simulink model "Redresseur_MLI_3Ph_MLI_antiwindup_sign"  (R2018b)
settings: Solver=ode8  StartTime=0.0  StopTime=Ts  FixedStep=1e-6  RelTol=1e-3
undefined symbols (not defined in the file): C, Im, inverter_matrix, K, L, R, Ta, Td, Ti, V
libraries: simulink x1
settings Model: Creator=driss  LastModifiedBy=driss
settings DataIOCC: ReturnWorkspaceOutputs=on
settings DebuggingCC: UnconnectedInputMsg=none  UnconnectedOutputMsg=none  UnconnectedLineMsg=none
settings ModelReferenceCC: EnableRefExpFcnMdlSchedulingChecks=off
settings RTWCC: Description=Generic Real-Time Target

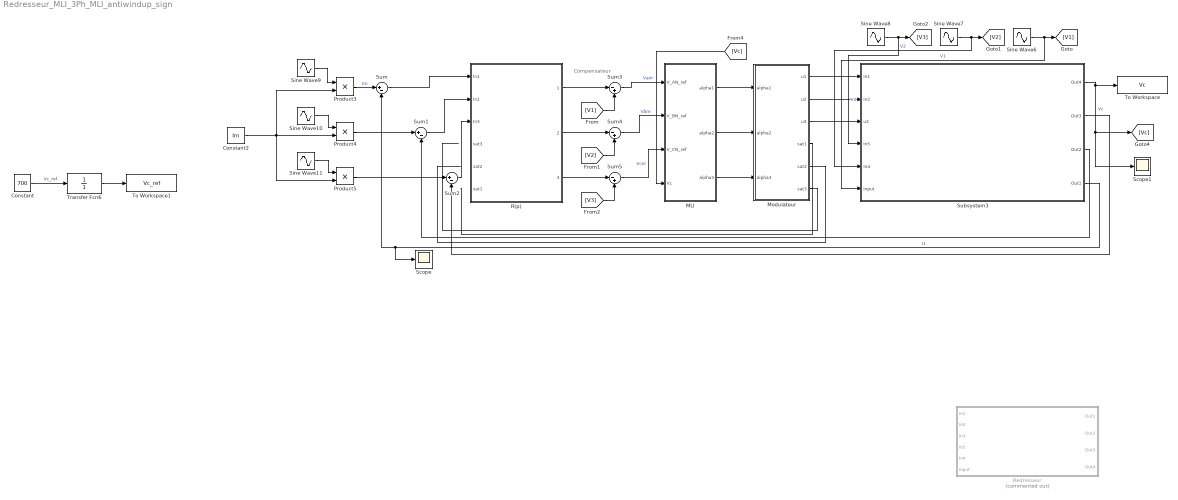
== system Redresseur_MLI_3Ph_MLI_antiwindup_sign ==
  note: Compensateur
  Constant : Constant  Value=700
  Constant2 : Constant  Value=Im
  MLI : Subsystem
  Modulateur : Subsystem
  Product3 : Product
  Product4 : Product
  Product5 : Product
  R(p) : Subsystem
  Redresseur : Subsystem  Commented=on
  Scope : Scope
  Scope1 : Scope
  Sine Wave10 : Sin  Frequency=2*50*pi  Phase=-2*pi/3  SampleTime=0
  Sine Wave11 : Sin  Frequency=2*50*pi  Phase=-4*pi/3  SampleTime=0
  Sine Wave6 : Sin  Amplitude=V*sqrt(2)  Frequency=2*50*pi  SampleTime=0
  Sine Wave7 : Sin  Amplitude=V*sqrt(2)  Frequency=2*50*pi  Phase=-2*pi/3  SampleTime=0
  Sine Wave8 : Sin  Amplitude=V*sqrt(2)  Frequency=2*50*pi  Phase=-4*pi/3  SampleTime=0
  Sine Wave9 : Sin  Frequency=2*50*pi  SampleTime=0
  Subsystem3 : Subsystem
  Sum : Sum  Inputs=|+-
  Sum1 : Sum  Inputs=|+-
  Sum2 : Sum  Inputs=|+-
  Sum3 : Sum  Inputs=|-+
  Sum4 : Sum  Inputs=|-+
  Sum5 : Sum  Inputs=|-+
  To Workspace : ToWorkspace  VariableName=Vc  SaveFormat=Timeseries  SampleTime=-1
  To Workspace1 : ToWorkspace  VariableName=Vc_ref  SaveFormat=Timeseries  SampleTime=-1
  Transfer Fcn6 : TransferFcn  Denominator=[0 1]
  wires:
  Constant/1 -> Transfer Fcn6/1  "Vc_ref"
  MLI/2(alpha2) -> Modulateur/2(alpha2)
  MLI/3(alpha3) -> Modulateur/3(alpha3)
  Modulateur/1(u1) -> Subsystem3/1(In1)
  Modulateur/2(u2) -> Subsystem3/2(In2)
  Modulateur/3(u3) -> Subsystem3/3(u3)
  Sine Wave7/1 -> [V2], Subsystem3/5(In4)  "V2"
  Sine Wave8/1 -> Subsystem3/4(In5), [V3]  "V3"
  Sine Wave6/1 -> [V1], Subsystem3/6(Input)  "V1"
  [Vc] -> MLI/4(Vc)
  Subsystem3/1(Out4) -> Scope1/1, [Vc], To Workspace/1  "Vc"
  Sine Wave11/1 -> Product5/1
  Sine Wave10/1 -> Product4/1
  Sine Wave9/1 -> Product3/1
  Constant2/1 -> Product5/2, Product4/2, Product3/2
  Product3/1 -> Sum/1  "Im"
  Product4/1 -> Sum1/1
  Product5/1 -> Sum2/1
  Subsystem3/2(Out3) -> Sum2/2
  Subsystem3/3(Out2) -> Sum1/2
  Subsystem3/4(Out1) -> Scope/1, Sum/2  "I1"
  Transfer Fcn6/1 -> To Workspace1/1
  Sum/1 -> R(p)/1(In1)
  Sum1/1 -> R(p)/2(In2)
  Sum2/1 -> R(p)/3(In3)
  R(p)/1(1) -> Sum3/1
  Sum3/1 -> MLI/1(V_AN_ref)  "Vanr"
  [V2] -> Sum4/2
  Sum4/1 -> MLI/2(V_BN_ref)  "Vbnr"
  R(p)/2(2) -> Sum4/1
  [V3] -> Sum5/2
  Sum5/1 -> MLI/3(V_CN_ref)  "Vcnr"
  R(p)/3(3) -> Sum5/1
  MLI/1(alpha1) -> Modulateur/1(alpha1)
  [V1] -> Sum3/2
  Modulateur/4(sat1) -> ?
  Modulateur/5(sat2) -> ?
  Modulateur/6(sat3) -> ?

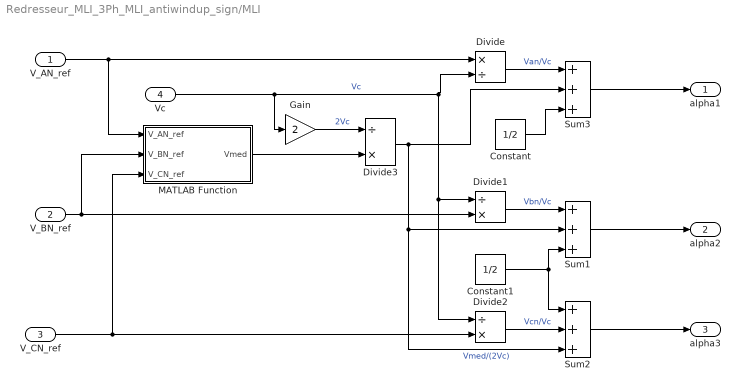
== system Redresseur_MLI_3Ph_MLI_antiwindup_sign/MLI ==
  V_AN_ref : Inport
  V_BN_ref : Inport  Port=2
  V_CN_ref : Inport  Port=3
  Vc : Inport  Port=4
  Constant : Constant  Value=1/2
  Constant1 : Constant  Value=1/2
  Divide : Product  Inputs=*/
  Divide1 : Product  Inputs=/*
  Divide2 : Product  Inputs=/*
  Divide3 : Product  Inputs=/*
  Gain : Gain  Gain=2
  MATLAB Function : MATLAB Function  TreatAsAtomicUnit=on
  Sum1 : Sum  Inputs=+++
  Sum2 : Sum  Inputs=+++
  Sum3 : Sum  Inputs=+++
  alpha1 : Outport  VectorParamsAs1DForOutWhenUnconnected=on
  alpha2 : Outport  Port=2  VectorParamsAs1DForOutWhenUnconnected=on
  alpha3 : Outport  Port=3  VectorParamsAs1DForOutWhenUnconnected=on
  wires:
  Sum3/1 -> alpha1/1
  V_AN_ref/1 -> MATLAB Function/1(V_AN_ref), Divide/1
  Divide/1 -> Sum3/1  "Van/Vc"
  Constant/1 -> Sum3/3
  MATLAB Function/1(Vmed) -> Divide3/2
  Gain/1 -> Divide3/1  "2Vc"
  Constant1/1 -> Sum2/1, Sum1/3
  Sum1/1 -> alpha2/1
  Divide1/1 -> Sum1/1  "Vbn/Vc"
  V_BN_ref/1 -> MATLAB Function/2(V_BN_ref), Divide1/2
  Divide3/1 -> Sum2/3, Sum1/2, Sum3/2  "Vmed/(2Vc)"
  Vc/1 -> Divide/2, Divide2/1, Divide1/1, Gain/1  "Vc"
  V_CN_ref/1 -> Divide2/2, MATLAB Function/3(V_CN_ref)
  Divide2/1 -> Sum2/2  "Vcn/Vc"
  Sum2/1 -> alpha3/1

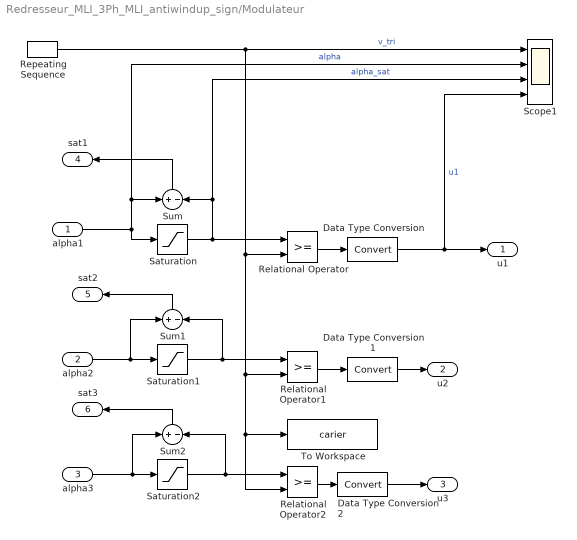
== system Redresseur_MLI_3Ph_MLI_antiwindup_sign/Modulateur ==
  alpha1 : Inport
  alpha2 : Inport  Port=2
  alpha3 : Inport  Port=3
  Data Type Conversion : DataTypeConversion
  Data Type Conversion1 : DataTypeConversion
  Data Type Conversion2 : DataTypeConversion
  Relational Operator : RelationalOperator  OutDataTypeStr=boolean  RndMeth=Simplest
  Relational Operator1 : RelationalOperator  OutDataTypeStr=boolean  RndMeth=Simplest
  Relational Operator2 : RelationalOperator  OutDataTypeStr=boolean  RndMeth=Simplest
  Repeating Sequence : simulink/Sources/Repeating Sequence  rep_seq_t=[0 Td/2 Td]  rep_seq_y=[1 0 1]
  Saturation : Saturate  UpperLimit=1  LowerLimit=0
  Saturation1 : Saturate  UpperLimit=1  LowerLimit=0
  Saturation2 : Saturate  UpperLimit=1  LowerLimit=0
  Scope1 : Scope  NumInputPorts=4
  Sum : Sum  Inputs=+-
  Sum1 : Sum  Inputs=+-
  Sum2 : Sum  Inputs=+-
  To Workspace : ToWorkspace  VariableName=carier  SaveFormat=Timeseries  SampleTime=-1
  u1 : Outport  VectorParamsAs1DForOutWhenUnconnected=on
  u2 : Outport  Port=2  VectorParamsAs1DForOutWhenUnconnected=on
  u3 : Outport  Port=3  VectorParamsAs1DForOutWhenUnconnected=on
  sat1 : Outport  Port=4  VectorParamsAs1DForOutWhenUnconnected=on
  sat2 : Outport  Port=5  VectorParamsAs1DForOutWhenUnconnected=on
  sat3 : Outport  Port=6  VectorParamsAs1DForOutWhenUnconnected=on
  wires:
  Relational Operator/1 -> Data Type Conversion/1
  alpha1/1 -> Saturation/1, Scope1/2, Sum/1  "alpha"
  Relational Operator1/1 -> Data Type Conversion1/1
  Relational Operator2/1 -> Data Type Conversion2/1
  Repeating Sequence/1 -> Relational Operator1/2, To Workspace/1, Relational Operator2/2, Relational Operator/2, Scope1/1  "v_tri"
  Saturation/1 -> Scope1/3, Sum/2, Relational Operator/1  "alpha_sat"
  Data Type Conversion/1 -> Scope1/4, u1/1  "u1"
  Data Type Conversion1/1 -> u2/1
  Data Type Conversion2/1 -> u3/1
  Sum/1 -> sat1/1
  Sum1/1 -> sat2/1
  Saturation1/1 -> Sum1/2, Relational Operator1/1
  alpha2/1 -> Sum1/1, Saturation1/1
  alpha3/1 -> Sum2/1, Saturation2/1
  Saturation2/1 -> Sum2/2, Relational Operator2/1
  Sum2/1 -> sat3/1

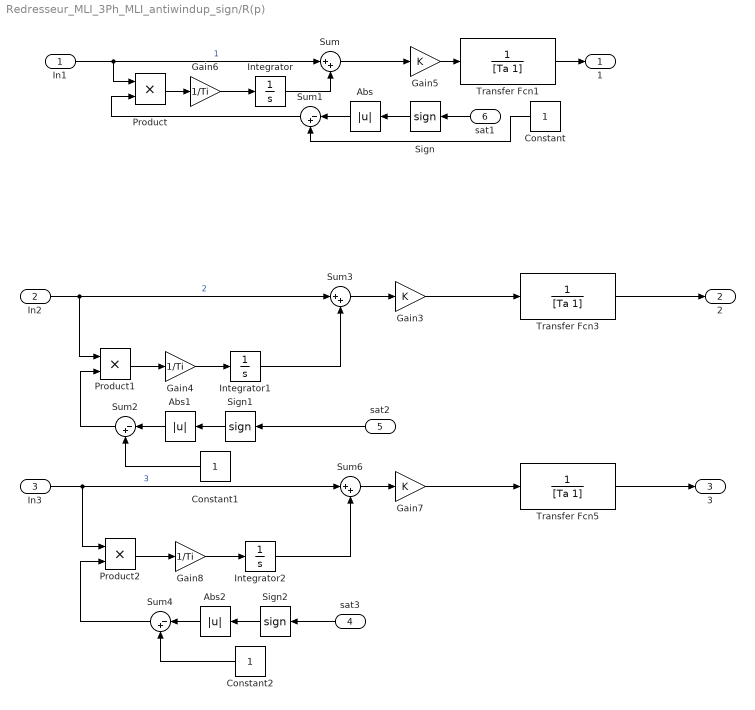
== system Redresseur_MLI_3Ph_MLI_antiwindup_sign/R(p) ==
  In1 : Inport
  In2 : Inport  Port=2
  In3 : Inport  Port=3
  sat3 : Inport  Port=4
  sat2 : Inport  Port=5
  sat1 : Inport  Port=6
  Abs : Abs
  Abs1 : Abs
  Abs2 : Abs
  Constant : Constant
  Constant1 : Constant
  Constant2 : Constant
  Gain3 : Gain  Gain=K
  Gain4 : Gain  Gain=1/Ti
  Gain5 : Gain  Gain=K
  Gain6 : Gain  Gain=1/Ti
  Gain7 : Gain  Gain=K
  Gain8 : Gain  Gain=1/Ti
  Integrator : Integrator  InitialCondition=1
  Integrator1 : Integrator  InitialCondition=1
  Integrator2 : Integrator
  Product : Product
  Product1 : Product
  Product2 : Product
  Sign : Signum
  Sign1 : Signum
  Sign2 : Signum
  Sum : Sum  Inputs=|++
  Sum1 : Sum  Inputs=|-+
  Sum2 : Sum  Inputs=|-+
  Sum3 : Sum  Inputs=|++
  Sum4 : Sum  Inputs=|-+
  Sum6 : Sum  Inputs=|++
  Transfer Fcn1 : TransferFcn  Denominator=[Ta 1]
  Transfer Fcn3 : TransferFcn  Denominator=[Ta 1]
  Transfer Fcn5 : TransferFcn  Denominator=[Ta 1]
  1 : Outport  VectorParamsAs1DForOutWhenUnconnected=on
  2 : Outport  Port=2  VectorParamsAs1DForOutWhenUnconnected=on
  3 : Outport  Port=3  VectorParamsAs1DForOutWhenUnconnected=on
  wires:
  Abs1/1 -> Sum2/1
  Product2/1 -> Gain8/1
  Sum/1 -> Gain5/1
  Product/1 -> Gain6/1
  Sum6/1 -> Gain7/1
  Sum2/1 -> Product1/2
  Sum4/1 -> Product2/2
  Sum3/1 -> Gain3/1
  Constant2/1 -> Sum4/2
  Product1/1 -> Gain4/1
  Sign2/1 -> Abs2/1
  Gain4/1 -> Integrator1/1
  Constant/1 -> Sum1/2
  Sum1/1 -> Product/2
  sat3/1 -> Sign2/1
  Abs2/1 -> Sum4/1
  Integrator/1 -> Sum/2
  Integrator2/1 -> Sum6/2
  Gain7/1 -> Transfer Fcn5/1
  Sign/1 -> Abs/1
  sat2/1 -> Sign1/1
  Constant1/1 -> Sum2/2
  Integrator1/1 -> Sum3/2
  Gain3/1 -> Transfer Fcn3/1
  sat1/1 -> Sign/1
  Gain5/1 -> Transfer Fcn1/1
  Gain8/1 -> Integrator2/1
  Sign1/1 -> Abs1/1
  Transfer Fcn3/1 -> 2/1
  Gain6/1 -> Integrator/1
  In2/1 -> Sum3/1, Product1/1  "2"
  Transfer Fcn1/1 -> 1/1
  Abs/1 -> Sum1/1
  In3/1 -> Sum6/1, Product2/1  "3"
  In1/1 -> Sum/1, Product/1  "1"
  Transfer Fcn5/1 -> 3/1

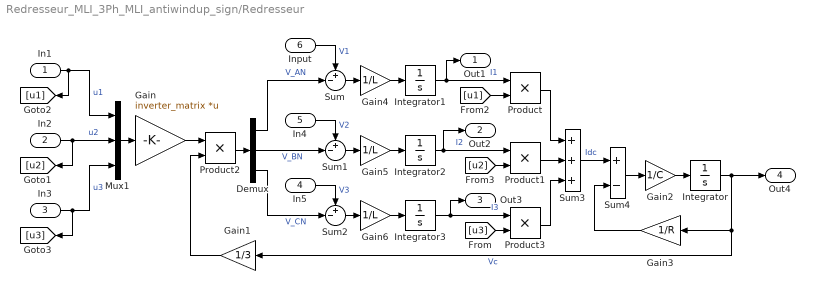
== system Redresseur_MLI_3Ph_MLI_antiwindup_sign/Redresseur ==
  In1 : Inport
  In2 : Inport  Port=2
  In3 : Inport  Port=3
  In5 : Inport  Port=4
  In4 : Inport  Port=5
  Input : Inport  Port=6
  Demux : Demux  Outputs=3
  Gain : Gain  Gain=inverter_matrix  Multiplication=Matrix(K*u)
  Gain1 : Gain  Gain=1/3
  Gain2 : Gain  Gain=1/C
  Gain3 : Gain  Gain=1/R
  Gain4 : Gain  Gain=1/L
  Gain5 : Gain  Gain=1/L
  Gain6 : Gain  Gain=1/L
  Integrator{,1..3} (4 alike) : Integrator
  Mux1 : Mux  Inputs=3
  Product{,1..3} (4 alike) : Product
  Sum : Sum  Inputs=+-|
  Sum1 : Sum  Inputs=+-|
  Sum2 : Sum  Inputs=+-|
  Sum3 : Sum  Inputs=+++
  Sum4 : Sum  Inputs=+-
  Out1 : Outport  VectorParamsAs1DForOutWhenUnconnected=on
  Out2 : Outport  Port=2  VectorParamsAs1DForOutWhenUnconnected=on
  Out3 : Outport  Port=3  VectorParamsAs1DForOutWhenUnconnected=on
  Out4 : Outport  Port=4  VectorParamsAs1DForOutWhenUnconnected=on
  wires:
  In3/1 -> [u3], Mux1/3  "u3"
  In2/1 -> [u2], Mux1/2  "u2"
  In1/1 -> [u1], Mux1/1  "u1"
  Demux/2 -> Sum1/2  "V_BN"
  Demux/3 -> Sum2/2  "V_CN"
  Demux/1 -> Sum/2  "V_AN"
  Input/1 -> Sum/1  "V1"
  In4/1 -> Sum1/1  "V2"
  In5/1 -> Sum2/1  "V3"
  Sum/1 -> Gain4/1
  Sum1/1 -> Gain5/1
  Sum2/1 -> Gain6/1
  Integrator1/1 -> Out1/1, Product/1  "I1"
  Integrator3/1 -> Out3/1, Product3/1  "I3"
  Integrator2/1 -> Product1/1, Out2/1  "I2"
  Mux1/1 -> Gain/1
  [u3] -> Product3/2
  Product/1 -> Sum3/1
  Product1/1 -> Sum3/2
  Product3/1 -> Sum3/3
  Gain1/1 -> Product2/2
  Gain/1 -> Product2/1
  Sum3/1 -> Sum4/1  "Idc"
  Sum4/1 -> Gain2/1
  Gain2/1 -> Integrator/1
  Integrator/1 -> Out4/1, Gain1/1, Gain3/1  "Vc"
  Gain3/1 -> Sum4/2
  Gain4/1 -> Integrator1/1
  Gain5/1 -> Integrator2/1
  Gain6/1 -> Integrator3/1
  Product2/1 -> Demux/1
  [u1] -> Product/2
  [u2] -> Product1/2

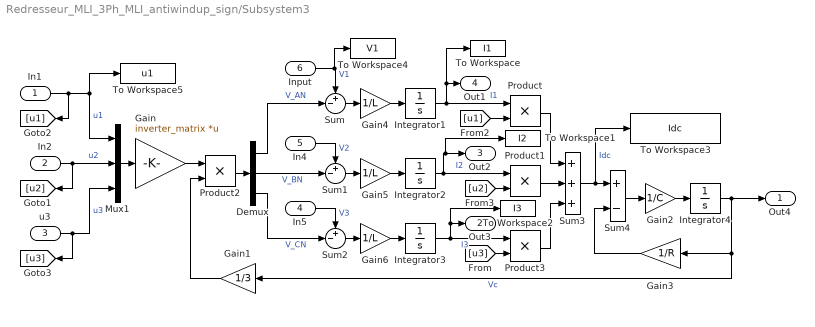
== system Redresseur_MLI_3Ph_MLI_antiwindup_sign/Subsystem3 ==
  In1 : Inport
  In2 : Inport  Port=2
  u3 : Inport  Port=3
  In5 : Inport  Port=4
  In4 : Inport  Port=5
  Input : Inport  Port=6
  Demux : Demux  Outputs=3
  Gain : Gain  Gain=inverter_matrix  Multiplication=Matrix(K*u)
  Gain1 : Gain  Gain=1/3
  Gain2 : Gain  Gain=1/C
  Gain3 : Gain  Gain=1/R
  Gain4 : Gain  Gain=1/L
  Gain5 : Gain  Gain=1/L
  Gain6 : Gain  Gain=1/L
  Integrator1 : Integrator
  Integrator2 : Integrator
  Integrator3 : Integrator
  Integrator4 : Integrator  InitialCondition=V*sqrt(2)*sqrt(3)
  Mux1 : Mux  Inputs=3
  Product{,1..3} (4 alike) : Product
  Sum : Sum  Inputs=+-|
  Sum1 : Sum  Inputs=+-|
  Sum2 : Sum  Inputs=+-|
  Sum3 : Sum  Inputs=+++
  Sum4 : Sum  Inputs=+-
  To Workspace : ToWorkspace  VariableName=I1  SaveFormat=Timeseries  SampleTime=-1
  To Workspace1 : ToWorkspace  VariableName=I2  SaveFormat=Timeseries  SampleTime=-1
  To Workspace2 : ToWorkspace  VariableName=I3  SaveFormat=Timeseries  SampleTime=-1
  To Workspace3 : ToWorkspace  VariableName=Idc  SaveFormat=Timeseries  SampleTime=-1
  To Workspace4 : ToWorkspace  VariableName=V1  SaveFormat=Timeseries  SampleTime=-1
  To Workspace5 : ToWorkspace  VariableName=u1  SaveFormat=Timeseries  SampleTime=-1
  Out4 : Outport  VectorParamsAs1DForOutWhenUnconnected=on
  Out3 : Outport  Port=2  VectorParamsAs1DForOutWhenUnconnected=on
  Out2 : Outport  Port=3  VectorParamsAs1DForOutWhenUnconnected=on
  Out1 : Outport  Port=4  VectorParamsAs1DForOutWhenUnconnected=on
  wires:
  [u2] -> Product1/2
  [u1] -> Product/2
  Product2/1 -> Demux/1
  Gain6/1 -> Integrator3/1
  Gain5/1 -> Integrator2/1
  Gain4/1 -> Integrator1/1
  Gain3/1 -> Sum4/2
  Integrator4/1 -> Gain3/1, Gain1/1, Out4/1  "Vc"
  Gain2/1 -> Integrator4/1
  Sum4/1 -> Gain2/1
  Sum3/1 -> Sum4/1, To Workspace3/1  "Idc"
  Gain/1 -> Product2/1
  Gain1/1 -> Product2/2
  Product3/1 -> Sum3/3
  Product1/1 -> Sum3/2
  Product/1 -> Sum3/1
  [u3] -> Product3/2
  Mux1/1 -> Gain/1
  Integrator2/1 -> Out2/1, To Workspace1/1, Product1/1  "I2"
  Integrator3/1 -> Product3/1, Out3/1, To Workspace2/1  "I3"
  Integrator1/1 -> Product/1, Out1/1, To Workspace/1  "I1"
  Sum2/1 -> Gain6/1
  Sum1/1 -> Gain5/1
  Sum/1 -> Gain4/1
  In5/1 -> Sum2/1  "V3"
  In4/1 -> Sum1/1  "V2"
  Input/1 -> Sum/1, To Workspace4/1  "V1"
  Demux/1 -> Sum/2  "V_AN"
  Demux/3 -> Sum2/2  "V_CN"
  Demux/2 -> Sum1/2  "V_BN"
  In1/1 -> To Workspace5/1, Mux1/1, [u1]  "u1"
  In2/1 -> Mux1/2, [u2]  "u2"
  u3/1 -> Mux1/3, [u3]  "u3"

== matlab function Redresseur_MLI_3Ph_MLI_antiwindup_sign/MLI/MATLAB Function ==
  data: V_AN_ref input; Vmed output; V_BN_ref input; V_CN_ref input
function Vmed = fcn(V_AN_ref,V_BN_ref,V_CN_ref)
     V_set = [V_AN_ref V_BN_ref V_CN_ref];
Vmed= -(min(V_set) + max(V_set));
